simulink model "test_supervisor"  (R2024b)
settings: Solver=FixedStepAuto  StartTime=0.0  StopTime=inf  RelTol=1e-3
undefined symbols (not defined in the file): ControlModes, EventTypes, InitConfParams, MotionControlInitConf
libraries: simulink x1
settings Model: DataDictionary=embeddedBoard_common.sldd  SimulationMode=accelerator  Creator=mfussi  LastModifiedBy=mfussi
settings SolverCC: ConcurrentTasks=on  AutoInsertRateTranBlk=on
settings DataIOCC: SaveOutput=off  DSMLogging=off  SaveTime=off
settings OptimizationCC: SimCompilerOptimization=on
settings DebuggingCC: ParameterPrecisionLossMsg=none
settings ModelReferenceCC: SupportModelReferenceSimTargetCustomCode=on
settings SFSimCC: SimTargetLang=C++
settings RTWCC: GPUComputeCapability=3.5

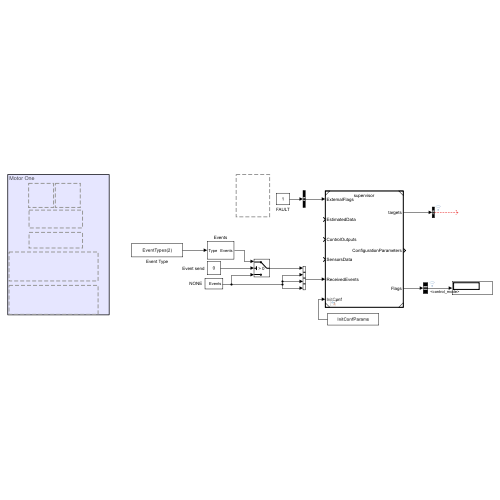
[thumbnail: Simulink's stored preview of the top-level diagram]
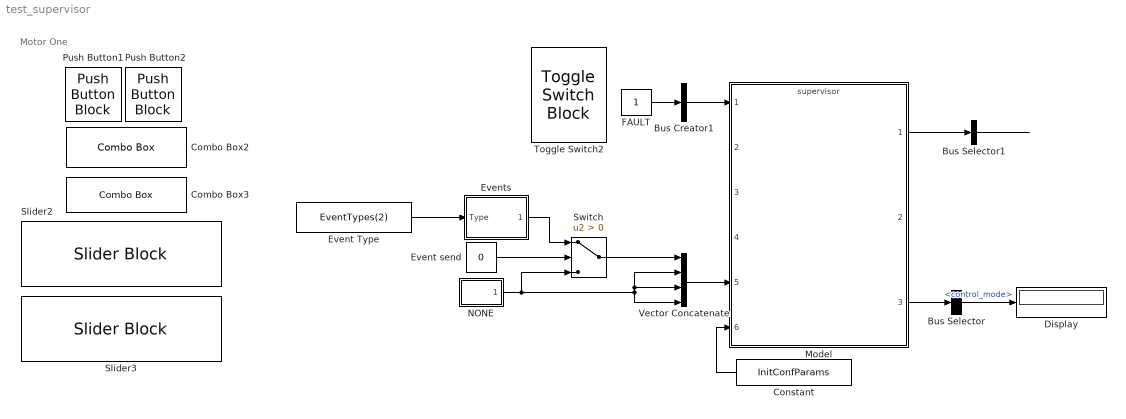
== system test_supervisor ==
  note: Motor One
  Bus Creator1 : BusCreator  Inputs=1  OutDataTypeStr=Bus: ExternalFlags  NonVirtualBus=on
      settings: InheritFromInputs=off
  Bus Selector : BusSelector  OutputSignals=control_mode
  Bus Selector1 : BusSelector  OutputSignals=motorcurrent  OutputAsBus=on
  Combo Box2 : ComboBox  SelectedLabel=SetControlMode  UseEnumeratedDataType=on  EnumeratedDataType=SupervisorEvents
      settings: Values={{'None', 'SetLimit', 'SetControlMode', 'SetMotorConfig', 'SetPid', 'SetTarget'}, [0 1 2 5 3 4]}
  Combo Box3 : ComboBox  SelectedLabel=Current  UseEnumeratedDataType=on  EnumeratedDataType=ControlModes
      settings: Values={{'NotConfigured', 'Idle', 'Position', 'PositionDirect', 'Current', 'Velocity', 'Voltage', 'Torque', 'HwFaultCM'}, [0 1 2 3 4 5 6 7 8]}
  Constant : Constant  Value=InitConfParams  OutDataTypeStr=Bus: ActuatorConfiguration  SampleTime=1e-3
  Display : Display
  Event Type : Constant  Value=EventTypes(2)  OutDataTypeStr=Enum: EventTypes
  Event send : Constant  Value=0
  Events : Subsystem
  FAULT : Constant  OutDataTypeStr=Inherit: Inherit via back propagation
  Model : ModelReference  ModelNameDialog=supervisor  SimulationMode=Normal  ModelReferenceVersion=3.2
  NONE : Subsystem
  Push Button1 : PushButtonBlock  ButtonText=Send  OffValue=0.000000
  Push Button2 : PushButtonBlock  ButtonText=Latch  ButtonType=Latch  OffValue=0.000000
  Slider2 : SliderBlock  ScaleMax=1
  Slider3 : SliderBlock  ScaleMax=0.36
  Switch : Switch  Criteria=u2 > Threshold  SaturateOnIntegerOverflow=off  InputSameDT=off
  Toggle Switch2 : ToggleSwitchBlock
      settings: Values={{'Off', 'On'}, [0 1]}
  Vector Concatenate : Concatenate  NumInputs=4
  wires:
  Event send/1 -> Switch/2
  Model/3 -> Bus Selector/1
  Model/1 -> Bus Selector1/1
  Bus Creator1/1 -> Model/1
  Constant/1 -> Model/6
  Switch/1 -> Vector Concatenate/1
  FAULT/1 -> Bus Creator1/1
  NONE/1(Events) -> Vector Concatenate/4, Vector Concatenate/3, Vector Concatenate/2, Switch/3
  Events/1(Events) -> Switch/1
  Vector Concatenate/1 -> Model/5
  Bus Selector/1 -> Display/1  "<control_mode>"
  Bus Selector1/1 -> ?
  Event Type/1 -> Events/1(Type)

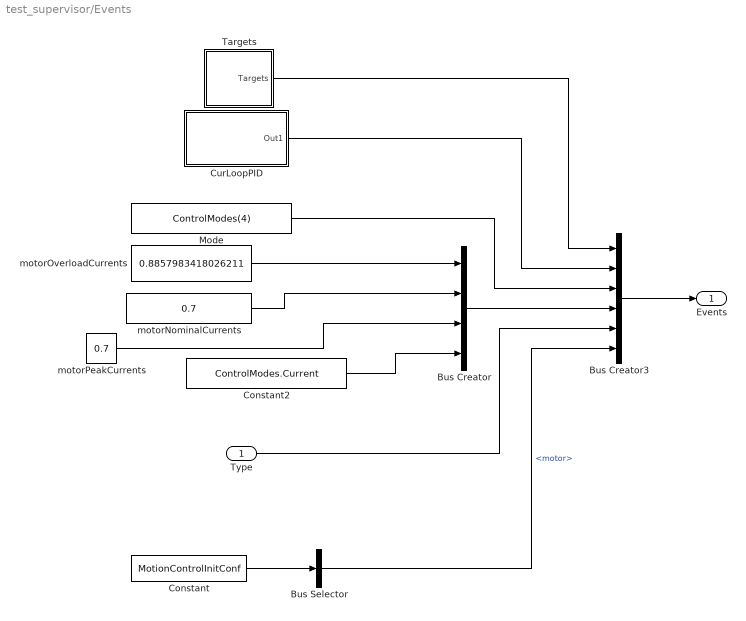
== system test_supervisor/Events ==
  Type : Inport
  Bus Creator : BusCreator  Inputs=4  OutDataTypeStr=Bus: SupervisorInputLimits  NonVirtualBus=on
      settings: InheritFromInputs=off
  Bus Creator3 : BusCreator  Inputs=6  OutDataTypeStr=Bus: SupervisorReceivedEvents  NonVirtualBus=on
      settings: InheritFromInputs=off
  Bus Selector : BusSelector  OutputSignals=motor
  Constant : Constant  Value=MotionControlInitConf  OutDataTypeStr=Bus: ActuatorConfiguration
  Constant2 : Constant  Value=ControlModes.Current  OutDataTypeStr=Enum: ControlModes
  CurLoopPID : Subsystem  mask{OutMax=0, OutMin=0, P=2, I=500, D=0, N=10, I0=0, D0=0, shift_factor=0}
      mask prompts: shift_factor "Shift Factor"
  Mode : Constant  Value=ControlModes(4)  OutDataTypeStr=Enum: ControlModes
  Targets : Subsystem
  motorNominalCurrents : Constant  Value=0.7  OutDataTypeStr=single
  motorOverloadCurrents : Constant  Value=0.8857983418026211  OutDataTypeStr=single
  motorPeakCurrents : Constant  Value=0.7  OutDataTypeStr=single
  Events : Outport  OutDataTypeStr=Bus: SupervisorReceivedEvents
  wires:
  Bus Creator/1 -> Bus Creator3/4
  Bus Selector/1 -> Bus Creator3/6  "<motor>"
  Mode/1 -> Bus Creator3/3
  Targets/1(Targets) -> Bus Creator3/1
  Type/1 -> Bus Creator3/5
  CurLoopPID/1(Out1) -> Bus Creator3/2
  motorPeakCurrents/1 -> Bus Creator/3
  Constant2/1 -> Bus Creator/4
  motorOverloadCurrents/1 -> Bus Creator/1
  motorNominalCurrents/1 -> Bus Creator/2
  Bus Creator3/1 -> Events/1
  Constant/1 -> Bus Selector/1

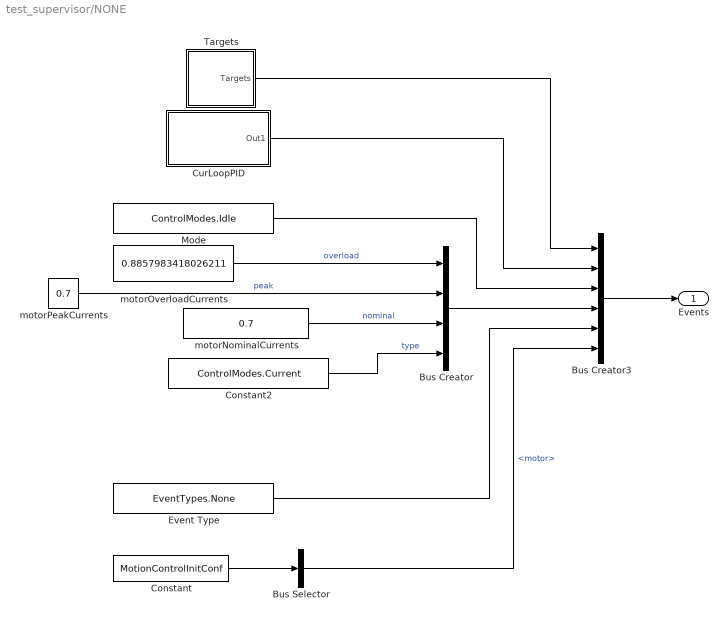
== system test_supervisor/NONE ==
  Bus Creator : BusCreator  Inputs=4  OutDataTypeStr=Bus: SupervisorInputLimits
  Bus Creator3 : BusCreator  Inputs=6  OutDataTypeStr=Bus: SupervisorReceivedEvents  NonVirtualBus=on
      settings: InheritFromInputs=off
  Bus Selector : BusSelector  OutputSignals=motor
  Constant : Constant  Value=MotionControlInitConf  OutDataTypeStr=Bus: ActuatorConfiguration
  Constant2 : Constant  Value=ControlModes.Current  OutDataTypeStr=Enum: ControlModes
  CurLoopPID : Subsystem  mask{OutMax=0, OutMin=0, P=2, I=500, D=0, N=10, I0=0, D0=0, shift_factor=0}
      mask prompts: shift_factor "Shift Factor"
  Event Type : Constant  Value=EventTypes.None  OutDataTypeStr=Enum: EventTypes
  Mode : Constant  Value=ControlModes.Idle  OutDataTypeStr=Enum: ControlModes
  Targets : Subsystem
  motorNominalCurrents : Constant  Value=0.7  OutDataTypeStr=single
  motorOverloadCurrents : Constant  Value=0.8857983418026211  OutDataTypeStr=single
  motorPeakCurrents : Constant  Value=0.7  OutDataTypeStr=single
  Events : Outport  OutDataTypeStr=Bus: SupervisorReceivedEvents
  wires:
  Bus Creator/1 -> Bus Creator3/4
  Bus Selector/1 -> Bus Creator3/6  "<motor>"
  Mode/1 -> Bus Creator3/3
  Targets/1(Targets) -> Bus Creator3/1
  Event Type/1 -> Bus Creator3/5
  CurLoopPID/1(Out1) -> Bus Creator3/2
  motorPeakCurrents/1 -> Bus Creator/2  "peak"
  Constant2/1 -> Bus Creator/4  "type"
  motorOverloadCurrents/1 -> Bus Creator/1  "overload"
  motorNominalCurrents/1 -> Bus Creator/3  "nominal"
  Bus Creator3/1 -> Events/1
  Constant/1 -> Bus Selector/1

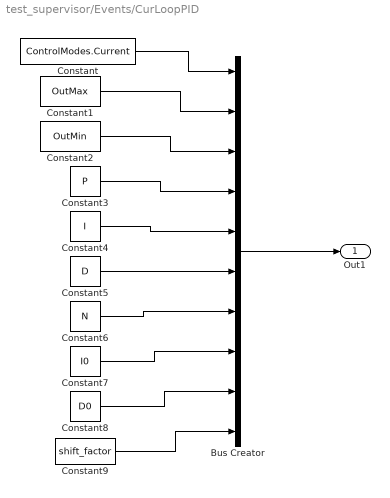
== system test_supervisor/Events/CurLoopPID ==
  Bus Creator : BusCreator  Inputs=10  OutDataTypeStr=Bus: PID  NonVirtualBus=on
      settings: InheritFromInputs=off
  Constant : Constant  Value=ControlModes.Current
  Constant1 : Constant  Value=OutMax  OutDataTypeStr=single
  Constant2 : Constant  Value=OutMin  OutDataTypeStr=single
  Constant3 : Constant  Value=P  OutDataTypeStr=single
  Constant4 : Constant  Value=I  OutDataTypeStr=single
  Constant5 : Constant  Value=D  OutDataTypeStr=single
  Constant6 : Constant  Value=N  OutDataTypeStr=single
  Constant7 : Constant  Value=I0  OutDataTypeStr=single
  Constant8 : Constant  Value=D0  OutDataTypeStr=single
  Constant9 : Constant  Value=shift_factor  OutDataTypeStr=uint8
  Out1 : Outport  OutDataTypeStr=Bus: PID
  wires:
  Bus Creator/1 -> Out1/1
  Constant8/1 -> Bus Creator/9
  Constant3/1 -> Bus Creator/4
  Constant5/1 -> Bus Creator/6
  Constant1/1 -> Bus Creator/2
  Constant7/1 -> Bus Creator/8
  Constant2/1 -> Bus Creator/3
  Constant9/1 -> Bus Creator/10
  Constant4/1 -> Bus Creator/5
  Constant/1 -> Bus Creator/1
  Constant6/1 -> Bus Creator/7

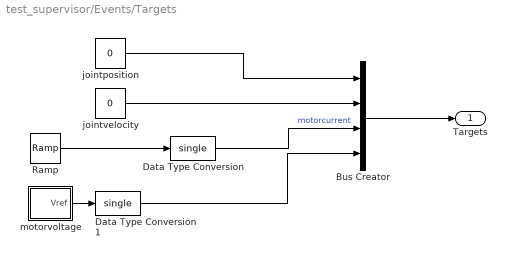
== system test_supervisor/Events/Targets ==
  Bus Creator : BusCreator  Inputs=4  OutDataTypeStr=Bus: Targets  NonVirtualBus=on
      settings: InheritFromInputs=off
  Data Type Conversion : DataTypeConversion  OutDataTypeStr=single  SaturateOnIntegerOverflow=off  RndMeth=Floor
  Data Type Conversion1 : DataTypeConversion  OutDataTypeStr=single  SaturateOnIntegerOverflow=off  RndMeth=Floor
  Ramp : simulink/Sources/Ramp  slope=0.01  start=0  InitialOutput=0
  jointposition : Constant  Value=0  OutDataTypeStr=single
  jointvelocity : Constant  Value=0  OutDataTypeStr=single
  motorvoltage : Subsystem
  Targets : Outport
  wires:
  Bus Creator/1 -> Targets/1
  jointposition/1 -> Bus Creator/1
  jointvelocity/1 -> Bus Creator/2
  Data Type Conversion1/1 -> Bus Creator/4
  Data Type Conversion/1 -> Bus Creator/3  "motorcurrent"
  motorvoltage/1(Vref) -> Data Type Conversion1/1
  Ramp/1 -> Data Type Conversion/1

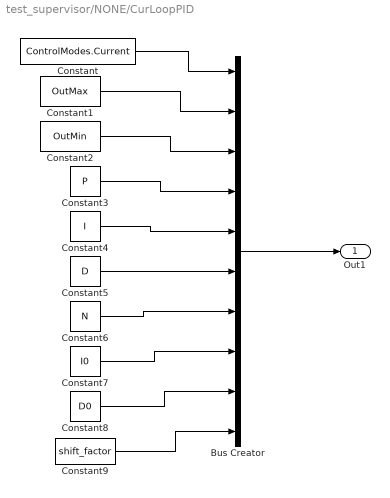
== system test_supervisor/NONE/CurLoopPID ==
  Bus Creator : BusCreator  Inputs=10  OutDataTypeStr=Bus: PID  NonVirtualBus=on
      settings: InheritFromInputs=off
  Constant : Constant  Value=ControlModes.Current
  Constant1 : Constant  Value=OutMax  OutDataTypeStr=single
  Constant2 : Constant  Value=OutMin  OutDataTypeStr=single
  Constant3 : Constant  Value=P  OutDataTypeStr=single
  Constant4 : Constant  Value=I  OutDataTypeStr=single
  Constant5 : Constant  Value=D  OutDataTypeStr=single
  Constant6 : Constant  Value=N  OutDataTypeStr=single
  Constant7 : Constant  Value=I0  OutDataTypeStr=single
  Constant8 : Constant  Value=D0  OutDataTypeStr=single
  Constant9 : Constant  Value=shift_factor  OutDataTypeStr=uint8
  Out1 : Outport  OutDataTypeStr=Bus: PID
  wires:
  Bus Creator/1 -> Out1/1
  Constant8/1 -> Bus Creator/9
  Constant3/1 -> Bus Creator/4
  Constant5/1 -> Bus Creator/6
  Constant1/1 -> Bus Creator/2
  Constant7/1 -> Bus Creator/8
  Constant2/1 -> Bus Creator/3
  Constant9/1 -> Bus Creator/10
  Constant4/1 -> Bus Creator/5
  Constant/1 -> Bus Creator/1
  Constant6/1 -> Bus Creator/7

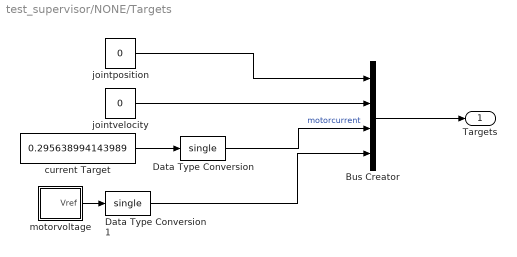
== system test_supervisor/NONE/Targets ==
  Bus Creator : BusCreator  Inputs=4  OutDataTypeStr=Bus: Targets  NonVirtualBus=on
      settings: InheritFromInputs=off
  Data Type Conversion : DataTypeConversion  OutDataTypeStr=single  SaturateOnIntegerOverflow=off  RndMeth=Floor
  Data Type Conversion1 : DataTypeConversion  OutDataTypeStr=single  SaturateOnIntegerOverflow=off  RndMeth=Floor
  current Target : Constant  Value=0.295638994143989
  jointposition : Constant  Value=0  OutDataTypeStr=single
  jointvelocity : Constant  Value=0  OutDataTypeStr=single
  motorvoltage : Subsystem
  Targets : Outport
  wires:
  Bus Creator/1 -> Targets/1
  jointposition/1 -> Bus Creator/1
  jointvelocity/1 -> Bus Creator/2
  Data Type Conversion1/1 -> Bus Creator/4
  Data Type Conversion/1 -> Bus Creator/3  "motorcurrent"
  motorvoltage/1(Vref) -> Data Type Conversion1/1
  current Target/1 -> Data Type Conversion/1

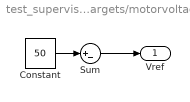
== system test_supervisor/Events/Targets/motorvoltage ==
  Constant : Constant  Value=50
  Sum : Sum  Inputs=|+-
  Vref : Outport
  wires:
  Sum/1 -> Vref/1
  Constant/1 -> Sum/1

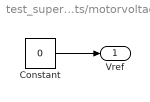
== system test_supervisor/NONE/Targets/motorvoltage ==
  Constant : Constant  Value=0
  Vref : Outport
  wires:
  Constant/1 -> Vref/1
